simulink model "ReactionWheel"  (R2018a)
settings: Solver=VariableStepAuto  StartTime=0.0  StopTime=10.0  RelTol=1e-3
values from neighbouring files (symbols this model uses):
  B_coef = 0.02    [BLDC.m]
  J = 0.00284    [BLDC.m]
  L = 2.72e-3    (= 0.00272)    [BLDC.m]
  lamda = 0.105    [BLDC.m]
  M = 1.5e-3    (= 0.0015)    [BLDC.m]
  P = 4    [BLDC.m]
  R = 0.75    [BLDC.m]
libraries: simulink x9, simulink_extras x3
settings Model: Creator=Siddharth Deore  LastModifiedBy=Siddharth Deore

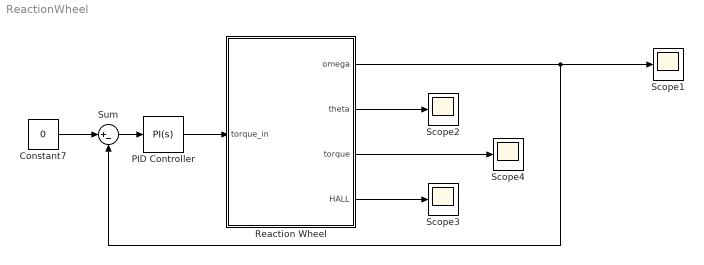
== system ReactionWheel ==
  Constant7 : Constant  Value=0
  PID Controller : simulink/Continuous/PID Controller  Controller=PI  TimeDomain=Continuous-time  SampleTime=-1  IntegratorMethod=Forward Euler  FilterMethod=Forward Euler  Form=Parallel  UseFilter=on  ControllerParametersSource=internal  P=2  I=5  D=0  N=100  InitialConditionSource=internal  InitialConditionForIntegrator=0  InitialConditionForFilter=0  ExternalReset=none  LimitOutput=off  UpperSaturationLimit=inf  LowerSaturationLimit=-inf  LinearizeAsGain=on  AntiWindupMode=none  Kb=1  TrackingMode=off  Kt=1  PParamMin=[]  PParamMax=[]  IParamMin=[]  IParamMax=[]  DParamMin=[]  DParamMax=[]  NParamMin=[]  NParamMax=[]  KbParamMin=[]  KbParamMax=[]  KtParamMin=[]  KtParamMax=[]  POutMin=[]  POutMax=[]  IOutMin=[]  IOutMax=[]  DOutMin=[]  DOutMax=[]  NOutMin=[]  NOutMax=[]  KbOutMin=[]  KbOutMax=[]  KtOutMin=[]  KtOutMax=[]  IntegratorOutMin=[]  IntegratorOutMax=[]  FilterOutMin=[]  FilterOutMax=[]  SumOutMin=[]  SumOutMax=[]  SumI1OutMin=[]  SumI1OutMax=[]  SumI2OutMin=[]  SumI2OutMax=[]  SumI3OutMin=[]  SumI3OutMax=[]  SumDOutMin=[]  SumDOutMax=[]  SaturationOutMin=[]  SaturationOutMax=[]  IntegratorContinuousStateAttributes=''  IntegratorStateMustResolveToSignalObject=off  IntegratorRTWStateStorageClass=Auto  FilterContinuousStateAttributes=''  FilterStateMustResolveToSignalObject=off  FilterRTWStateStorageClass=Auto  DifferentiatorICPrevScaledInput=0  DifferentiatorOutMin=[]  DifferentiatorOutMax=[]  FilterDiffOutCoefMin=[]  FilterDiffOutCoefMax=[]  SumDenOutMin=[]  SumDenOutMax=[]  SumNumOutMin=[]  SumNumOutMax=[]  ReciprocalOutMin=[]  ReciprocalOutMax=[]  DivideOutMin=[]  DivideOutMax=[]  TunerSelectOption=Transfer Function Based (PID Tuner App)
  Reaction Wheel : Subsystem
  Scope{1..4} (4 alike) : Scope
  Sum : Sum  Inputs=|+-
  wires:
  Sum/1 -> PID Controller/1
  Constant7/1 -> Sum/1
  Reaction Wheel/1(omega) -> Scope1/1, Sum/2
  PID Controller/1 -> Reaction Wheel/1(torque_in)
  Reaction Wheel/2(theta) -> Scope2/1
  Reaction Wheel/3(torque) -> Scope4/1
  Reaction Wheel/4(HALL) -> Scope3/1

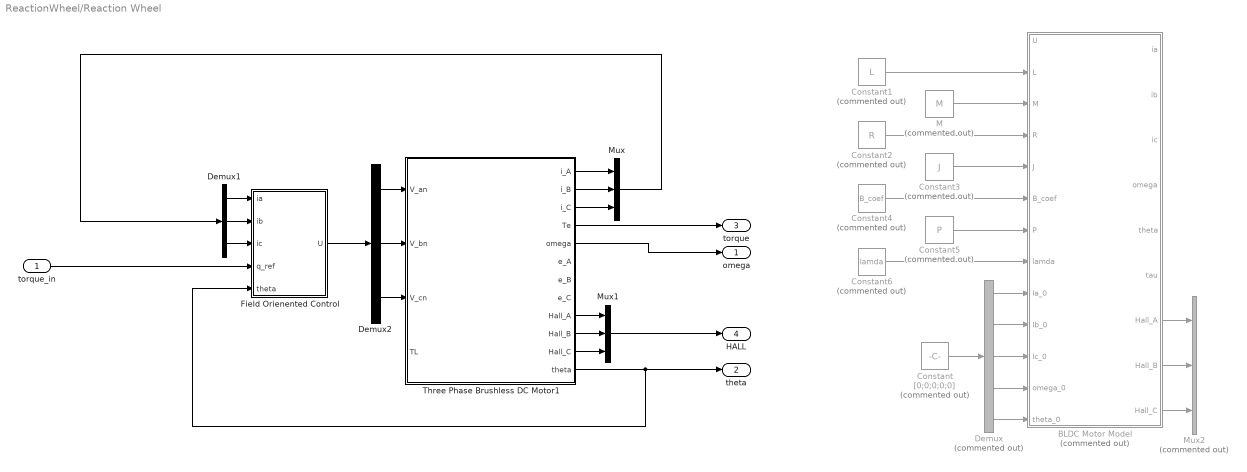
== system ReactionWheel/Reaction Wheel ==
  torque_in : Inport
  BLDC Motor Model : Subsystem  Commented=on
  Constant : Constant  Commented=on  Value=[0;0;0;0;0]
  Constant1 : Constant  Commented=on  Value=L
  Constant2 : Constant  Commented=on  Value=R
  Constant3 : Constant  Commented=on  Value=J
  Constant4 : Constant  Commented=on  Value=B_coef
  Constant5 : Constant  Commented=on  Value=P
  Constant6 : Constant  Commented=on  Value=lamda
  Demux : Demux  Commented=on  Outputs=5
  Demux1 : Demux  Outputs=3
  Demux2 : Demux  Outputs=3
  Field Orienented Control : Subsystem
  M : Constant  Commented=on  Value=M
  Mux : Mux  Inputs=3
  Mux1 : Mux  Inputs=3
  Mux2 : Mux  Commented=on  Inputs=3
  Three Phase Brushless DC Motor1 : Subsystem  mask{B=0.000052, J=0.0007, Ke=0.0071, Kt=0.0071, L=0.005, P=4, R=3.25}
      mask prompts: B "Viscous damping"; J "Innertia"; Ke "Back-EMF constant"; Kt "Torque constant"; L "Mutual Inductance"; P "Number of Pole Pairs"; R "Coil Resistance"
  omega : Outport
  theta : Outport  Port=2
  torque : Outport  Port=3
  HALL : Outport  Port=4
  wires:
  Three Phase Brushless DC Motor1/3(i_C) -> Mux/3
  Three Phase Brushless DC Motor1/9(Hall_A) -> Mux1/1
  Constant/1 -> Demux/1
  Three Phase Brushless DC Motor1/11(Hall_C) -> Mux1/3
  Three Phase Brushless DC Motor1/1(i_A) -> Mux/1
  Three Phase Brushless DC Motor1/2(i_B) -> Mux/2
  Mux1/1 -> HALL/1
  Demux1/3 -> Field Orienented Control/3(ic)
  Three Phase Brushless DC Motor1/12(theta) -> theta/1, Field Orienented Control/5(theta)
  Mux/1 -> Demux1/1
  Field Orienented Control/1(U) -> Demux2/1
  Demux/1 -> BLDC Motor Model/9(Ia_0)
  Demux/2 -> BLDC Motor Model/10(Ib_0)
  Three Phase Brushless DC Motor1/10(Hall_B) -> Mux1/2
  Demux1/1 -> Field Orienented Control/1(ia)
  Demux1/2 -> Field Orienented Control/2(ib)
  Three Phase Brushless DC Motor1/4(Te) -> torque/1
  Demux/3 -> BLDC Motor Model/11(Ic_0)
  Demux/4 -> BLDC Motor Model/12(omega_0)
  Demux/5 -> BLDC Motor Model/13(theta_0)
  Three Phase Brushless DC Motor1/5(omega) -> omega/1
  torque_in/1 -> Field Orienented Control/4(q_ref)
  Constant2/1 -> BLDC Motor Model/4(R)
  Constant1/1 -> BLDC Motor Model/2(L)
  Constant5/1 -> BLDC Motor Model/7(P)
  Constant6/1 -> BLDC Motor Model/8(lamda)
  M/1 -> BLDC Motor Model/3(M)
  Constant3/1 -> BLDC Motor Model/5(J)
  Constant4/1 -> BLDC Motor Model/6(B_coef)
  Demux2/3 -> Three Phase Brushless DC Motor1/3(V_cn)
  Demux2/1 -> Three Phase Brushless DC Motor1/1(V_an)
  Demux2/2 -> Three Phase Brushless DC Motor1/2(V_bn)
  BLDC Motor Model/8(Hall_B) -> Mux2/2
  BLDC Motor Model/7(Hall_A) -> Mux2/1
  BLDC Motor Model/9(Hall_C) -> Mux2/3

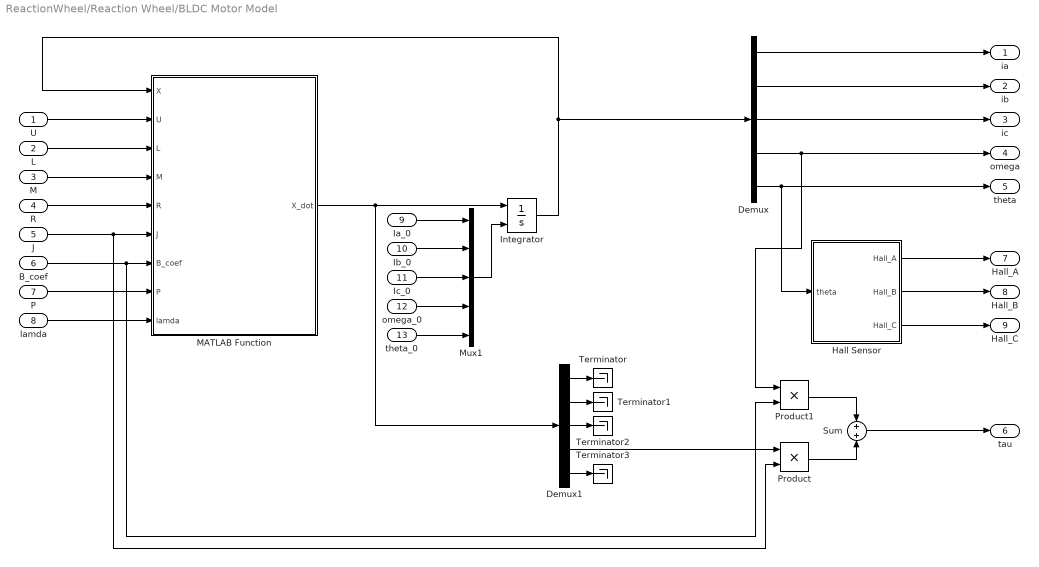
== system ReactionWheel/Reaction Wheel/BLDC Motor Model ==
  U : Inport
  L : Inport  Port=2
  M : Inport  Port=3
  R : Inport  Port=4
  J : Inport  Port=5
  B_coef : Inport  Port=6
  P : Inport  Port=7
  lamda : Inport  Port=8
  Ia_0 : Inport  Port=9
  Ib_0 : Inport  Port=10
  Ic_0 : Inport  Port=11
  omega_0 : Inport  Port=12
  theta_0 : Inport  Port=13
  Demux : Demux  Outputs=5
  Demux1 : Demux  Outputs=5
  Hall Sensor : Subsystem
  Integrator : Integrator  InitialConditionSource=external  InitialCondition=[0;0;0;0;0]
  MATLAB Function : MATLAB Function  TreatAsAtomicUnit=on
  Mux1 : Mux  Inputs=5
  Product : Product
  Product1 : Product
  Sum : Sum
  Terminator{,1..3} (4 alike) : Terminator
  ia : Outport
  ib : Outport  Port=2
  ic : Outport  Port=3
  omega : Outport  Port=4
  theta : Outport  Port=5
  tau : Outport  Port=6
  Hall_A : Outport  Port=7
  Hall_B : Outport  Port=8
  Hall_C : Outport  Port=9
  wires:
  U/1 -> MATLAB Function/2(U)
  Ic_0/1 -> Mux1/3
  Ib_0/1 -> Mux1/2
  Hall Sensor/1(Hall_A) -> Hall_A/1
  Hall Sensor/2(Hall_B) -> Hall_B/1
  Ia_0/1 -> Mux1/1
  Demux/5 -> theta/1, Hall Sensor/1(theta)
  omega_0/1 -> Mux1/4
  Hall Sensor/3(Hall_C) -> Hall_C/1
  lamda/1 -> MATLAB Function/9(lamda)
  P/1 -> MATLAB Function/8(P)
  Mux1/1 -> Integrator/2
  Integrator/1 -> Demux/1, MATLAB Function/1(X)
  L/1 -> MATLAB Function/3(L)
  R/1 -> MATLAB Function/5(R)
  B_coef/1 -> Product1/2, MATLAB Function/7(B_coef)
  Demux/3 -> ic/1
  theta_0/1 -> Mux1/5
  Demux/1 -> ia/1
  Demux/2 -> ib/1
  MATLAB Function/1(X_dot) -> Integrator/1, Demux1/1
  Demux/4 -> Product1/1, omega/1
  J/1 -> Product/2, MATLAB Function/6(J)
  M/1 -> MATLAB Function/4(M)
  Demux1/4 -> Product/1
  Demux1/1 -> Terminator/1
  Demux1/2 -> Terminator1/1
  Demux1/3 -> Terminator2/1
  Demux1/5 -> Terminator3/1
  Product/1 -> Sum/2
  Product1/1 -> Sum/1
  Sum/1 -> tau/1

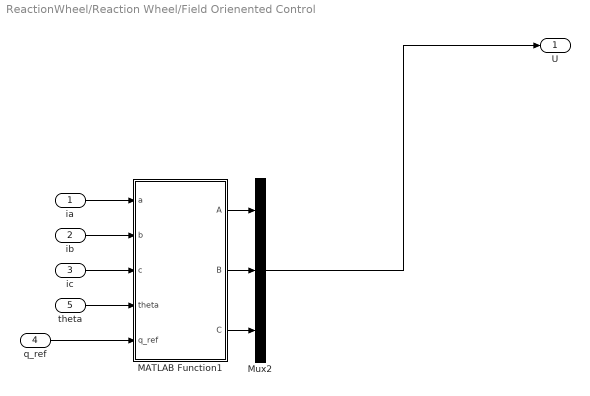
== system ReactionWheel/Reaction Wheel/Field Orienented Control ==
  ia : Inport
  ib : Inport  Port=2
  ic : Inport  Port=3
  q_ref : Inport  Port=4
  theta : Inport  Port=5
  MATLAB Function1 : MATLAB Function  TreatAsAtomicUnit=on
  Mux2 : Mux  Inputs=3
  U : Outport
  wires:
  MATLAB Function1/1(A) -> Mux2/1
  theta/1 -> MATLAB Function1/4(theta)
  ib/1 -> MATLAB Function1/2(b)
  MATLAB Function1/2(B) -> Mux2/2
  MATLAB Function1/3(C) -> Mux2/3
  Mux2/1 -> U/1
  q_ref/1 -> MATLAB Function1/5(q_ref)
  ia/1 -> MATLAB Function1/1(a)
  ic/1 -> MATLAB Function1/3(c)

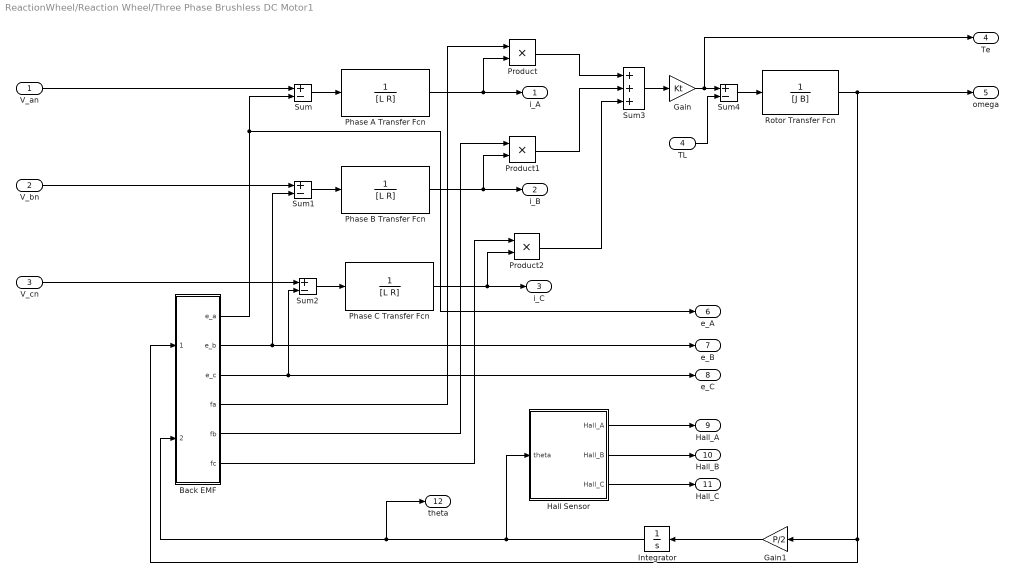
== system ReactionWheel/Reaction Wheel/Three Phase Brushless DC Motor1 ==
  V_an : Inport
  V_bn : Inport  Port=2
  V_cn : Inport  Port=3
  TL : Inport  Port=4
  Back EMF : Subsystem
  Gain : Gain  Gain=Kt
  Gain1 : Gain  Gain=P/2
  Hall Sensor : Subsystem
  Integrator : Integrator
  Phase A Transfer Fcn : TransferFcn  Denominator=[L R]
  Phase B Transfer Fcn : TransferFcn  Denominator=[L R]
  Phase C Transfer Fcn : TransferFcn  Denominator=[L R]
  Product : Product
  Product1 : Product
  Product2 : Product
  Rotor Transfer Fcn : TransferFcn  Denominator=[J B]
  Sum{,1..2,4} (4 alike) : Sum  Inputs=+-
  Sum3 : Sum  Inputs=+++
  i_A : Outport
  i_B : Outport  Port=2
  i_C : Outport  Port=3
  Te : Outport  Port=4
  omega : Outport  Port=5
  e_A : Outport  Port=6
  e_B : Outport  Port=7
  e_C : Outport  Port=8
  Hall_A : Outport  Port=9
  Hall_B : Outport  Port=10
  Hall_C : Outport  Port=11
  theta : Outport  Port=12
  wires:
  Integrator/1 -> theta/1, Back EMF/2(theta), Hall Sensor/1(theta)
  Back EMF/2(e_b) -> e_B/1, Sum1/2
  V_bn/1 -> Sum1/1
  Gain1/1 -> Integrator/1
  Product2/1 -> Sum3/3
  Rotor Transfer Fcn/1 -> omega/1, Back EMF/1(omega), Gain1/1
  Hall Sensor/2(Hall_B) -> Hall_B/1
  V_an/1 -> Sum/1
  Back EMF/6(fc) -> Product2/1
  Back EMF/3(e_c) -> e_C/1, Sum2/2
  Hall Sensor/3(Hall_C) -> Hall_C/1
  Back EMF/1(e_a) -> e_A/1, Sum/2
  Back EMF/5(fb) -> Product1/1
  Gain/1 -> Te/1, Sum4/1
  Sum2/1 -> Phase C Transfer Fcn/1
  Phase A Transfer Fcn/1 -> i_A/1, Product/2
  Back EMF/4(fa) -> Product/1
  Sum/1 -> Phase A Transfer Fcn/1
  Sum1/1 -> Phase B Transfer Fcn/1
  Phase C Transfer Fcn/1 -> i_C/1, Product2/2
  Product/1 -> Sum3/1
  Phase B Transfer Fcn/1 -> i_B/1, Product1/2
  Sum3/1 -> Gain/1
  V_cn/1 -> Sum2/1
  Product1/1 -> Sum3/2
  Hall Sensor/1(Hall_A) -> Hall_A/1
  TL/1 -> Sum4/2
  Sum4/1 -> Rotor Transfer Fcn/1

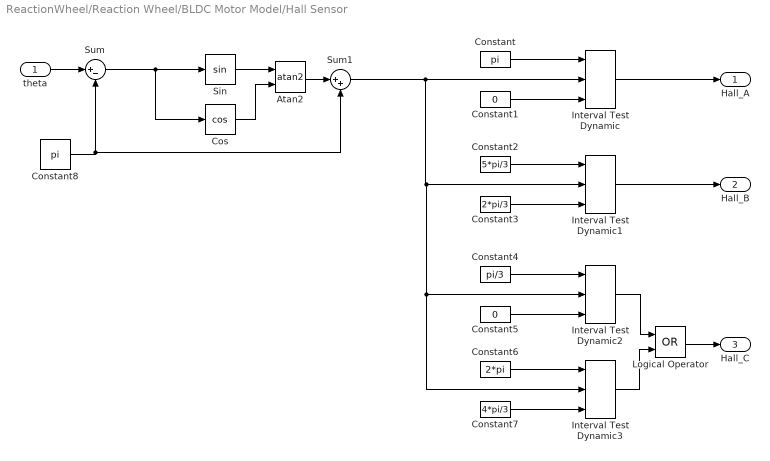
== system ReactionWheel/Reaction Wheel/BLDC Motor Model/Hall Sensor ==
  theta : Inport
  Atan2 : Trigonometry  Operator=atan2
  Constant : Constant  Value=pi
  Constant1 : Constant  Value=0
  Constant2 : Constant  Value=5*pi/3
  Constant3 : Constant  Value=2*pi/3
  Constant4 : Constant  Value=pi/3
  Constant5 : Constant  Value=0
  Constant6 : Constant  Value=2*pi
  Constant7 : Constant  Value=4*pi/3
  Constant8 : Constant  Value=pi
  Cos : Trigonometry  Operator=cos
  Interval Test Dynamic{,1..3} (4 alike) : simulink/Logic and Bit Operations/Interval Test Dynamic  IntervalClosedRight=on  IntervalClosedLeft=on  OutDataTypeStr=boolean
      settings: SourceProductName=Simulink  SourceProductBaseCode=SL
  Logical Operator : Logic  Operator=OR  AllPortsSameDT=off  OutDataTypeStr=boolean
  Sin : Trigonometry
  Sum : Sum  Inputs=|+-
  Sum1 : Sum  Inputs=|++
  Hall_A : Outport
  Hall_B : Outport  Port=2
  Hall_C : Outport  Port=3
  wires:
  Constant/1 -> Interval Test Dynamic/1
  Constant1/1 -> Interval Test Dynamic/3
  Constant3/1 -> Interval Test Dynamic1/3
  Constant2/1 -> Interval Test Dynamic1/1
  Constant5/1 -> Interval Test Dynamic2/3
  Constant4/1 -> Interval Test Dynamic2/1
  Constant7/1 -> Interval Test Dynamic3/3
  Constant6/1 -> Interval Test Dynamic3/1
  Interval Test Dynamic2/1 -> Logical Operator/1
  Interval Test Dynamic3/1 -> Logical Operator/2
  Logical Operator/1 -> Hall_C/1
  Interval Test Dynamic1/1 -> Hall_B/1
  Interval Test Dynamic/1 -> Hall_A/1
  Sin/1 -> Atan2/1
  Cos/1 -> Atan2/2
  theta/1 -> Sum/1
  Atan2/1 -> Sum1/1
  Sum/1 -> Cos/1, Sin/1
  Constant8/1 -> Sum1/2, Sum/2
  Sum1/1 -> Interval Test Dynamic3/2, Interval Test Dynamic2/2, Interval Test Dynamic1/2, Interval Test Dynamic/2

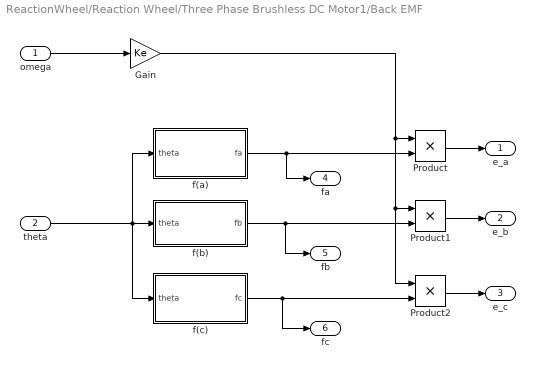
== system ReactionWheel/Reaction Wheel/Three Phase Brushless DC Motor1/Back EMF ==
  omega : Inport
  theta : Inport  Port=2
  Gain : Gain  Gain=Ke
  Product : Product
  Product1 : Product
  Product2 : Product
  f(a) : Subsystem
  f(b) : Subsystem
  f(c) : Subsystem
  e_a : Outport
  e_b : Outport  Port=2
  e_c : Outport  Port=3
  fa : Outport  Port=4
  fb : Outport  Port=5
  fc : Outport  Port=6
  wires:
  omega/1 -> Gain/1
  Product/1 -> e_a/1
  Product1/1 -> e_b/1
  Product2/1 -> e_c/1
  Gain/1 -> Product2/1, Product1/1, Product/1
  f(a)/1(fa) -> fa/1, Product/2
  f(b)/1(fb) -> fb/1, Product1/2
  f(c)/1(fc) -> fc/1, Product2/2
  theta/1 -> f(c)/1(theta), f(a)/1(theta), f(b)/1(theta)

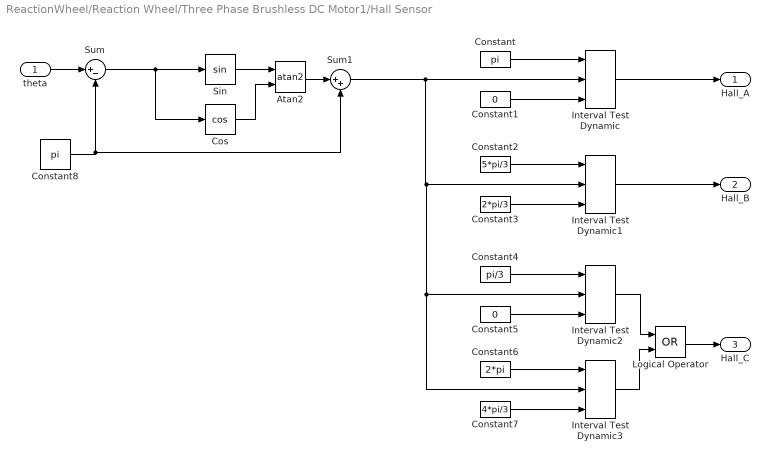
== system ReactionWheel/Reaction Wheel/Three Phase Brushless DC Motor1/Hall Sensor ==
  theta : Inport
  Atan2 : Trigonometry  Operator=atan2
  Constant : Constant  Value=pi
  Constant1 : Constant  Value=0
  Constant2 : Constant  Value=5*pi/3
  Constant3 : Constant  Value=2*pi/3
  Constant4 : Constant  Value=pi/3
  Constant5 : Constant  Value=0
  Constant6 : Constant  Value=2*pi
  Constant7 : Constant  Value=4*pi/3
  Constant8 : Constant  Value=pi
  Cos : Trigonometry  Operator=cos
  Interval Test Dynamic{,1..3} (4 alike) : simulink/Logic and Bit Operations/Interval Test Dynamic  IntervalClosedRight=on  IntervalClosedLeft=on  OutDataTypeStr=boolean
      settings: SourceProductName=Simulink  SourceProductBaseCode=SL
  Logical Operator : Logic  Operator=OR  AllPortsSameDT=off  OutDataTypeStr=boolean
  Sin : Trigonometry
  Sum : Sum  Inputs=|+-
  Sum1 : Sum  Inputs=|++
  Hall_A : Outport
  Hall_B : Outport  Port=2
  Hall_C : Outport  Port=3
  wires:
  Constant/1 -> Interval Test Dynamic/1
  Constant1/1 -> Interval Test Dynamic/3
  Constant3/1 -> Interval Test Dynamic1/3
  Constant2/1 -> Interval Test Dynamic1/1
  Constant5/1 -> Interval Test Dynamic2/3
  Constant4/1 -> Interval Test Dynamic2/1
  Constant7/1 -> Interval Test Dynamic3/3
  Constant6/1 -> Interval Test Dynamic3/1
  Interval Test Dynamic2/1 -> Logical Operator/1
  Interval Test Dynamic3/1 -> Logical Operator/2
  Logical Operator/1 -> Hall_C/1
  Interval Test Dynamic1/1 -> Hall_B/1
  Interval Test Dynamic/1 -> Hall_A/1
  Sin/1 -> Atan2/1
  Cos/1 -> Atan2/2
  theta/1 -> Sum/1
  Atan2/1 -> Sum1/1
  Sum/1 -> Cos/1, Sin/1
  Constant8/1 -> Sum1/2, Sum/2
  Sum1/1 -> Interval Test Dynamic3/2, Interval Test Dynamic2/2, Interval Test Dynamic1/2, Interval Test Dynamic/2

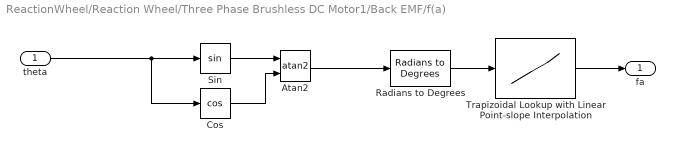
== system ReactionWheel/Reaction Wheel/Three Phase Brushless DC Motor1/Back EMF/f(a) ==
  theta : Inport
  Atan2 : Trigonometry  Operator=atan2
  Cos : Trigonometry  Operator=cos
  Radians to Degrees : simulink_extras/Transformations/Radians to Degrees
  Sin : Trigonometry
  Trapizoidal Lookup with Linear Point-slope Interpolation : Lookup_n-D  NumberOfTableDimensions=1  BreakpointsForDimension1="[-180,  -120,   -60,     0,    60,   120,   180]"  Table=[-1,-1,-1,1,1,1,-1]  InternalRulePriority=Speed  RndMeth=Simplest  InputSameDT=on
  fa : Outport
  wires:
  Trapizoidal Lookup with Linear Point-slope Interpolation/1 -> fa/1
  Cos/1 -> Atan2/2
  Sin/1 -> Atan2/1
  Radians to Degrees/1 -> Trapizoidal Lookup with Linear Point-slope Interpolation/1
  Atan2/1 -> Radians to Degrees/1
  theta/1 -> Cos/1, Sin/1

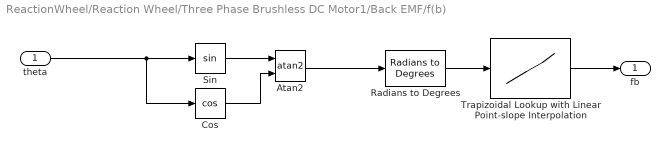
== system ReactionWheel/Reaction Wheel/Three Phase Brushless DC Motor1/Back EMF/f(b) ==
  theta : Inport
  Atan2 : Trigonometry  Operator=atan2
  Cos : Trigonometry  Operator=cos
  Radians to Degrees : simulink_extras/Transformations/Radians to Degrees
  Sin : Trigonometry
  Trapizoidal Lookup with Linear Point-slope Interpolation : Lookup_n-D  NumberOfTableDimensions=1  BreakpointsForDimension1="[-180,  -120,   -60,     0,    60,   120,   180]"  Table=[1,1,-1,-1,-1,1,1]  InternalRulePriority=Speed  RndMeth=Simplest  InputSameDT=on
  fb : Outport
  wires:
  Trapizoidal Lookup with Linear Point-slope Interpolation/1 -> fb/1
  Cos/1 -> Atan2/2
  Sin/1 -> Atan2/1
  Radians to Degrees/1 -> Trapizoidal Lookup with Linear Point-slope Interpolation/1
  Atan2/1 -> Radians to Degrees/1
  theta/1 -> Cos/1, Sin/1

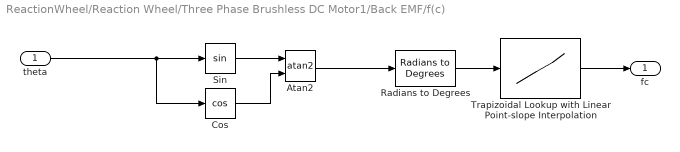
== system ReactionWheel/Reaction Wheel/Three Phase Brushless DC Motor1/Back EMF/f(c) ==
  theta : Inport
  Atan2 : Trigonometry  Operator=atan2
  Cos : Trigonometry  Operator=cos
  Radians to Degrees : simulink_extras/Transformations/Radians to Degrees
  Sin : Trigonometry
  Trapizoidal Lookup with Linear Point-slope Interpolation : Lookup_n-D  NumberOfTableDimensions=1  BreakpointsForDimension1="[-180,  -120,   -60,     0,    60,   120,   180]"  Table=[-1,1,1,1,-1,-1,-1]  InternalRulePriority=Speed  RndMeth=Simplest  InputSameDT=on
  fc : Outport
  wires:
  Trapizoidal Lookup with Linear Point-slope Interpolation/1 -> fc/1
  Cos/1 -> Atan2/2
  Sin/1 -> Atan2/1
  Radians to Degrees/1 -> Trapizoidal Lookup with Linear Point-slope Interpolation/1
  Atan2/1 -> Radians to Degrees/1
  theta/1 -> Cos/1, Sin/1

== matlab function ReactionWheel/Reaction Wheel/Field Orienented Control/MATLAB Function1 ==
  data: a input; A output; b input; c input; theta input; q_ref input; B output; C output
function [A,B,C] = foc(a,b,c,theta,q_ref)
    theta = theta - pi/2; % Phase correction for a alinged with q axis
    ct = cos(theta);
    st = sin(theta);
 
    % /*  Clarke Transform - abc to alpha beta */
    alpha = ((2*a) - b - c)/3;
    beta  = (b-c)*0.5773;
    % /* Clarke to Park Transform - alpha beta to dq */
    % // phase a alinged with q axis
    d = alpha*st - beta*ct;
    q = alpha*ct + beta*st;
    % // phase a aligned with d axis
    % d = alpha*ct + beta*st;
    % q =-alpha*st + beta*ct;
    
    % // flux PI Regulator
    d=0-d; 
    q=q_ref-q;
    % /* Park to Clarke Transform - alpha beta to dq */
    % // phase a alinged with q axis
    % alpha = d*st+q*ct; 
    % beta = -d*ct+q*st;
    % // phase a aligned with d axis
    alpha = d*ct-q*st; 
    beta =  d*st+q*ct;
    A =   alpha;
    B = - alpha*0.5 + 0.8661*beta; 
    C = - alpha*0.5 - 0.8661*beta;
%{
% Clarke a-b-c to alpha-beta
[alpha,beta]=clarke(a,b,c);

% Park alpha-beta to d-q
[d,q]=park(alpha,beta,theta);

% Torque PI Controller
q_err=(tau-q);
q_command = q_err*1; % PI

% inverse Park d-q to alpha-beta
[a,b] = inv_park(-d,-q_command,theta);

% inverse Clarke alpha-beta to a-b-c
[A,B,C] = inv_clarke(a,b);
end
function [alpha,beta]= clarke(a,b,c)
% abc to alpha beta
alpha = a;
beta =  0.5774*(a+2*b);
%}
end

== matlab function ReactionWheel/Reaction Wheel/BLDC Motor Model/MATLAB Function ==
  data: X input; X_dot output; U input; L input; M input; R input; J input; B_coef input; P input; lamda input
function X_dot = BLDCDynamics(X,U,L,M,R,J,B_coef,P,lamda)
%global integ_e
%% States
%{
i_a=X(1);       % current a [Amp]
i_b=X(2);       % current b [Amp]
i_c=X(3);       % current c [Amp]
%}
w = X(4);       % angular velocity [rad/sec]
theta = X(5);   % rotor angle [rad]
%{
% Motor Constants
L = 2.72e-3;        % self-inductance phase  (L_aa = L_bb = L_cc) [H]
M = 1.5e-3;         % mutual-inductance ( L_ab = L_bc = L_ca = M) [H]
Ls = L - M;         % [H]
R = 0.75;           % stator resistance per phase [ohm]
J = 0.00284;        % inertia [Kg-m/sec^2]
B_coef = 0.02;      % friction coefficient  [N-m/rad/sec]
P = 4;              % number of poles
lamda =  0.105;     % flux linkage wb
%}
Ls = L - M;         % [H]
%% sin back EMF
fa=sin(theta);
fb=sin(theta-2*pi/3);
fc=sin(theta+2*pi/3);
%% trapezoid back EMF
%[fa,fb,fc]=trapezoid(theta);

%% State Space
INV_Ls = 1/Ls;
INV_J = 1/J;
lfa=lamda*fa*INV_J;
lfb=lamda*fb*INV_J;
lfc=lamda*fc*INV_J;

A = [
        -R*INV_Ls,   0,  0,  lfa,  0;
        0,   -R*INV_Ls,  0,  lfb,  0;
        0,   0,  -R*INV_Ls,  lfc,  0;
        lfa, lfb, lfc,  -B_coef*INV_J, 0;
        0,  0,  0,  P/2,    0 ];
B = [
        INV_Ls,    0,  0,  0;
        0,    INV_Ls,  0,  0;
        0,    0,  INV_Ls,  0;
        0,    0,  0, INV_Ls;];
C = [
        -INV_Ls,0,0;
        0,-INV_Ls,0;
        0,0,-INV_Ls;
    ];

back_emf = w*lamda*[fa;fb;fc];
%%  PI Controller
%omega_e = 10-w;
%tau_command=(omega_e*1.5+integ_e*0.0009);
%integ_e=integ_e+omega_e;
%% field oriented control
%[VA,VB,VC]=foc(i_a,i_b,i_c,theta,tau_command);
%U = [VA;VB;VC;0];
%%
X_dot = A*X+[B*[U;0];0]+[C*back_emf;0;0];
%y = u;
